simulink model "UDP_Recieve"  (R2015a)
settings: Solver=ode45  StartTime=0.0  StopTime=inf  RelTol=1e-3
libraries: realtime_pacer_lib x2, etargetslib x1, dspnetwork x1
settings Model: SimulationMode=accelerator  Creator=dlwalter  LastModifiedBy=dlwalter

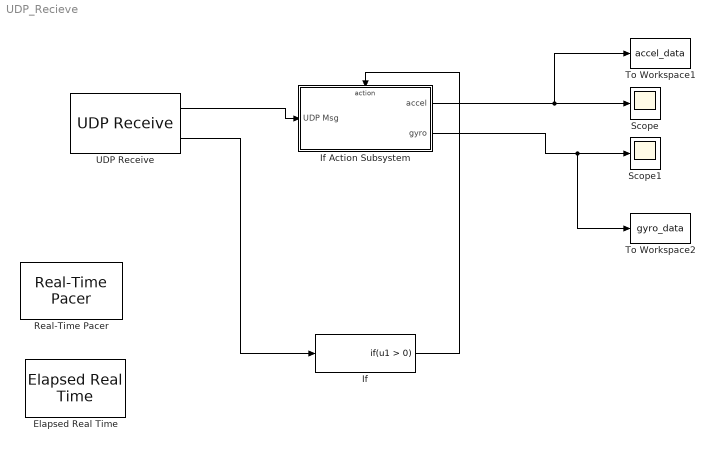
== system UDP_Recieve ==
  Elapsed Real Time : realtime_pacer_lib/Elapsed Real Time
  If : If  ShowElse=off  ZeroCross=off
  If Action Subsystem : Subsystem  TreatAsAtomicUnit=on
  Real-Time Pacer : realtime_pacer_lib/Real-Time Pacer  simTimePerRealTime=1
  Scope : Scope
      settings: YMin=-0.1  YMax=1.2
  Scope1 : Scope
      settings: YMin=-2.5  YMax=3.25
  To Workspace1 : ToWorkspace  VariableName=accel_data  SaveFormat=Timeseries  SampleTime=-1
  To Workspace2 : ToWorkspace  VariableName=gyro_data  SaveFormat=Timeseries  SampleTime=-1
  UDP Receive : dspnetwork/UDP Receive  localURL='0.0.0.0'  localPort=25001  remoteURL='169.254.1.10'  remotePort=-1  recvBufferSize=8192  dims=48  signalDatatype=uint8  isVarSize=off  showBlockingTime=on  blockingTime=.0001  sampletime=.001  blockPlatform=ZYNQ
  wires:
  UDP Receive/1 -> If Action Subsystem/1(UDP Msg)
  UDP Receive/2 -> If/1
  If/1 -> If Action Subsystem/Action
  If Action Subsystem/2(gyro) -> To Workspace2/1, Scope1/1
  If Action Subsystem/1(accel) -> To Workspace1/1, Scope/1

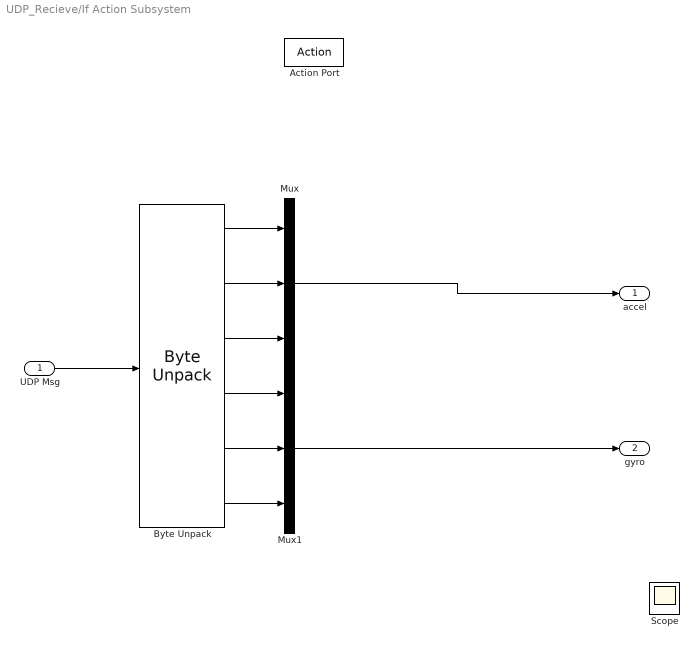
== system UDP_Recieve/If Action Subsystem ==
  UDP Msg : Inport
  Action Port : ActionPort  InitializeStates=reset  ActionType=then
  Byte Unpack : etargetslib/Byte Unpack  dimensions={1,1,1,1,1,1}  datatypes={'double','double','double','double','double','double'}  byteAlign=2
  Mux : Mux  Inputs=3
  Mux1 : Mux  Inputs=3
  Scope : Scope
      settings: SaveName=ScopeData2
  accel : Outport
  gyro : Outport  Port=2
  wires:
  Mux/1 -> accel/1
  UDP Msg/1 -> Byte Unpack/1
  Byte Unpack/1 -> Mux/1
  Byte Unpack/2 -> Mux/2
  Byte Unpack/3 -> Mux/3
  Byte Unpack/5 -> Mux1/2
  Byte Unpack/6 -> Mux1/3
  Byte Unpack/4 -> Mux1/1
  Mux1/1 -> gyro/1
